simulink model "Model2_V032_R_T4"  (R2023a)
settings: Solver=ode14x  StartTime=0.0  StopTime=Inf  FixedStep=ts  MaxStep=ts  RelTol=1e-5
values from neighbouring files (symbols this model uses):
  ausrollen_a_v = parameters.ausrollen_a_v    [efficiencycalc.m]    (also in parameters_initials.mat = 1)
  bremspunkte = parameters.bremspunkte    [efficiencycalc.m]    (also in parameters_initials.mat = [6100  280  8; 10400  500  3; 14100  550  8; 17729  0  1])
  brennstoffzellen_eta_kennfeld = parameters.brennstoffzellen_eta_kennfeld    [efficiencycalc.m]    (also in parameters_initials.mat = )
  brennstoffzellen_ui_kennfeld = parameters.brennstoffzellen_ui_kennfeld    [efficiencycalc.m]    (also in parameters_initials.mat = )
  coeffs_motor_moment = parameters.coeffs_motor_moment    [efficiencycalc.m]    (also in parameters_initials.mat = [30 30 30 5 7.5 10 0 0 0 6000 6000 6000 ... (30 elements, 3x)
  coeffs_motor_wirkungsgrad = parameters.coeffs_motor_wirkungsgrad    [efficiencycalc.m]    (also in parameters_initials.mat = [30 30 30 5 7.5 10 0 0 0 6000 6000 6000 ... (39 elements, 3x)
  fahrzeug_parameter = parameters.fahrzeug_parameter    [efficiencycalc.m]    (also in parameters_initials.mat = )
  strategie_parameter = parameters.strategie_parameter    [efficiencycalc.m]    (also in parameters_initials.mat = )
  strecke = parameters.strecke    [efficiencycalc.m]    (also in parameters_initials.mat = )
  ts = parameters.ts    [efficiencycalc.m]    (also in parameters_initials.mat = 0.01)
  U_moment = parameters.U_moment    [efficiencycalc.m]    (also in parameters_initials.mat = [30 3])
  U_wirkungsgrad = parameters.U_wirkungsgrad    [efficiencycalc.m]    (also in parameters_initials.mat = [30 3])
  umwelt_parameter = parameters.umwelt_parameter    [efficiencycalc.m]    (also in parameters_initials.mat = )
  zwangsgas = zeros(length(strecke.x),strecke.Rundenzahl)    [Automatisierung_Model_2.m]    (also in efficiencycalc.m; parameters_initials.mat = [0 0 0 0 0 0 0 0 0 0 0 0 ... (2563 elements, 233x11)])
libraries: simulink x1
(part 2 of 3)

== matlab function Model2_V032_R_T4/Energieversorgung/aktueller Ladestatus ==
  data: A_Status input; C_SC input; brennstoffzellen_ui_kennfeld_koeff input; brennstoffzellen_ui_kennfeld_min input; brennstoffzellen_ui_kennfeld_max input; end_charge_Zeitpuffer input; U_SC_initial input; U_SC input; A_Status_neu output; U_SC_min input; t_ges_zul input; Zeit input; ts input; Ladezeit output; v input; x_rest input; ende_bz_an input
function [ A_Status_neu , Ladezeit ]= fcn( A_Status , C_SC, brennstoffzellen_ui_kennfeld_koeff , brennstoffzellen_ui_kennfeld_min , brennstoffzellen_ui_kennfeld_max , end_charge_Zeitpuffer , U_SC_initial , U_SC, U_SC_min, t_ges_zul, Zeit , ts, v, x_rest , ende_bz_an)
%% Aktueller Ladestatus
% Hydro2Motion
% Prototyp: Homer
% Stand: 23.01.2020
% edited: Timo Freilinger

%% Eingang
% A_Status:                                 [-]     alter Status (aus vorherigem Zeitschritt): 0 nicht laden, 1 laden
% C_SC:                                     [F]     Kapazität der SuperCaps
% brennstoffzellen_ui_kennfeld_koeff:       [-]     Koeffizienten des Polynoms, welches Strom aus aktueller Spannung bestimmt
% brennstoffzellen_ui_kennfeld_min:         [V]     untere Spannungsgrenze, ab welcher das Polynom gültig ist
% brennstoffzellen_ui_kennfeld_max:         [V]     obere Spannungsgrenze, bis welcher das Polynom gültig ist
% end_charge_Zeitpuffer:                    [sec]   Zeitpuffer, um am Ende des Rennens früher als nötig begonnen wird, die SC auf Anfangsniveau zu laden (= Zeitunterschied zu Gesamtzeit, die erlaubt ist)
% U_SC_initial:                             [V]     Spannung SC zu Beginn des Rennens (= Spannung, welche am Ende des Rennens wieder vorhanden sein muss)
% U_SC:                                     [V]     aktuelle Spannung SC
% U_SC_min:                                 [V]     in fahrzeug_parameter festgelegte untere Grenze der Spannung SC
% t_ges_zul:                                [sec]   zulässige Gesamtzeit des Rennens
% Zeit:                                     [sec]   aktuelle Simulationszeit
% ts:                                       [sec]   Zeitintervall Berechnung
% v:                                        [m/s]   akt. Geschwindigkeit
% x_rest:                                   [m]     verbleibende Strecke


%% Ausgang
% A_Status_neu:                             [-]     neuer Status (1: Laden, 0: nicht Laden)
% Ladezeit:                                 [sec]   näherungsweise berechnete Zeit, die benötigt wird, um die SC von U_SC (aktuell) auf U_SC_initial zu laden (angenommen, es wird in dieser Zeit nicht zusätzlich Leistung entnommen)

%% Berechnung

%% Initialisierung
A_Status_neu = 0;
Ladezeit = 0;
delta_U = 0;
I_charge = 0;

%% Zeit, die zum Aufladen auf U_SC_initial benötigt werden würde
U_SC_help = U_SC;                                                                                   % U_SC_help: "Hilfsspannung", welche Aufladung symbolisiert
while U_SC_help <= U_SC_initial                                                                     % solange die Spannung kleiner als U_SC_initial ist
    % Berechnung aktueller Ladestrom aus aktueller Spannung (hilf)
    if U_SC_help < brennstoffzellen_ui_kennfeld_min                                            % wenn die aktuelle Spannung (hilf) kleiner als die untere Grenze des Polynoms ist
        I_charge = polyval(brennstoffzellen_ui_kennfeld_koeff,brennstoffzellen_ui_kennfeld_min);     % verwende die untere Grenze des Polynoms als Spannung zur Berechnung des Stroms
    elseif U_SC_help > brennstoffzellen_ui_kennfeld_max                                        % wenn die aktuelle Spannung (hilf) größer als die untere Grenze des Polynoms ist
        I_charge = polyval(brennstoffzellen_ui_kennfeld_koeff,brennstoffzellen_ui_kennfeld_max);     % verwende die obere Grenze des Polynoms als Spannung zur Berechnung des Stroms
    else                                                                                            % ansonsten
        I_charge = polyval(brennstoffzellen_ui_kennfeld_koeff,U_SC_help);                                 % verwende die aktuelle Spannung (hilf) zur Auswertung des Polynoms
    end
    % delta Spannung aus gerade vorliegendem Ladestrom berechnen
    delta_U = I_charge * 10 * ts / C_SC;                                                            % 10, da nur Annäherung! Es wird also angenommen, dass mit dem aktuellen Ladestrom 10*ts geladen wird (Diskretisierung).
    % neue Spannung (hilf) aus alter und delta berechnen
    U_SC_help = U_SC_help + delta_U;
    % Berechnung Ladezeit
    if Zeit ~= 0
        Ladezeit = Ladezeit + 10 * ts;
    end
end

%% Abfrage ob wegen Ende der Strecke nachgeladen wird
% Verbleibende Strecke --> Zeit berechnen mit akt. Geschwindigkeit --> mit
% Ladezeit vergleichen

% v = x / t --> t = x / v
if v > 0
    if x_rest / v - end_charge_Zeitpuffer <= Ladezeit                % Es wird geladen, sobald die restliche Zeit (mit Zeitpuffer) bis ins Ziel kleinergleich der benötigten Ladezeit ist
        A_Status_neu = 1;
    end
end

%% Einschalten BZ
% nach Kriterien:
if A_Status == 0 && U_SC < U_SC_min                              % Unterschreiten der unteren Grenze während Entladung
    A_Status_neu = 1;
elseif U_SC > U_SC_initial                                       % Überschreiten der oberen Grenze
    A_Status_neu = 0;
elseif A_Status == 1 && U_SC > U_SC_min && U_SC < U_SC_initial   % weiter Laden, wenn zwischen Grenzen und geladen wird
    A_Status_neu = 1;
elseif A_Status == 1 && U_SC < U_SC_min                          % falls das unmögliche möglich wird... (so hoher Spannungsabfall, dass kein Berechnungsschritt zwischen oberer und unterer Grenze)
    A_Status_neu = 1;
end

if ende_bz_an == 1
    A_Status_neu = 1;
end
end

== matlab function Model2_V032_R_T4/Energieversorgung/aktueller Ladestrom ==
  data: brennstoffzellen_ui_kennfeld_koeff input; brennstoffzellen_ui_kennfeld_min input; brennstoffzellen_ui_kennfeld_max input; U_SC input; I_charge output; A_Status input
function I_charge = fcn( brennstoffzellen_ui_kennfeld_koeff , brennstoffzellen_ui_kennfeld_min , brennstoffzellen_ui_kennfeld_max , U_SC , A_Status )
%% Aktueller Ladestrom
% Hydro2Motion
% Prototyp: Homer
% Stand: 23.01.2020
% edited: Timo Freilinger

%% Eingang
% brennstoffzellen_ui_kennfeld_koeff:       [-]     Koeffizienten des Polynoms, welches Strom aus aktueller Spannung bestimmt
% brennstoffzellen_ui_kennfeld_min:         [V]     untere Spannungsgrenze, ab welcher das Polynom gültig ist
% brennstoffzellen_ui_kennfeld_max:         [V]     obere Spannungsgrenze, bis welcher das Polynom gültig ist
% U_SC:                                     [V]     aktuelle Spannung SC
% A_Status:                                 [-]     aktueller Ladestatus (1: Laden, 0: nicht Laden)

%% Ausgang
% I_charge:                                 [A]     aktueller Ladestrom

%% Berechnung

% Initialisierung, bzw. Ladestrom, wenn nicht geladen wird
I_charge = 0;
% wenn geladen wird
if A_Status == 1
    % prüfen, ob aktuelle Spannung außerhalb der für das Polynom verwendeten Grezen liegt
    if U_SC > brennstoffzellen_ui_kennfeld_max                 % wenn die aktuelle Spannung größer als die obere Grenze des Polynoms ist
        U_SC = brennstoffzellen_ui_kennfeld_max;               % verwende die obere Grenze des Polynoms als Spannung zur Berechnung des Stroms
    elseif U_SC < brennstoffzellen_ui_kennfeld_min             % wenn die aktuelle Spannung kleiner als die untere Grenze des Polynoms ist
        U_SC = brennstoffzellen_ui_kennfeld_min;               % verwende die untere Grenze des Polynoms als Spannung zur Berechnung des Stroms
    end
    % berechne aktuellen Ladestrom, abhängig von der aktuellen Spannung
    I_charge = polyval(brennstoffzellen_ui_kennfeld_koeff, U_SC);
end

end

== matlab function Model2_V032_R_T4/Energieversorgung/Berechnung delta Spannung Aufladung ==
  data: I_charge input; ts input; C_SC input; delta_U_SC_charge output; t input
function delta_U_SC_charge = fcn( I_charge , ts , C_SC , t )
%% Berechnung delta Spannung Aufladung
% Hydro2Motion
% Prototyp: Homer
% Stand: 23.01.2020
% edited: Timo Freilinger

%% Eingang
% I_charge:             [A]     aktueller Ladestrom
% ts:                   [sec]   Zeitintervall Berechnung
% C_SC:                 [F]     Kapazität der Kondensatoren
% t:                    [sec]   aktuelle Simulationszeit

%% Ausgang
% delta_U_SC_charge:    [V]     aktuelle Spannungsdifferenz, mit der SC aufgeladen werden

%% Berechnung

if t == 0                                        % Initialisierung zu Beginn der Simulation
    delta_U_SC_charge = 0;
elseif I_charge == 0                             % wenn kein Ladestrom vorhanden
    delta_U_SC_charge = 0;                       % wird nicht geladen
else                                             % wenn Ladestrom vorhanden
    delta_U_SC_charge = I_charge * ts / C_SC;    % Spannungsdifferenz berechnen
end

end

== matlab function Model2_V032_R_T4/Fahr-Dynamik/Widerstände über Kennzahlen/Berechnung Luftwiderstand ==
  data: rho_0 input; F_L output; v input; cw_A input
function F_L = fcn(rho_0,v,cw_A)
%% Besrechnung Luftwiderstand
% Hydro2Motion
% Prototyp: Homer
% Stand: 04.01.2018
% edited: Robin Nedella, Timo Freilinger

%% Eingang
% rho_0:    [kg/m^3]    Luftdichte
% v:        [m/s]       aktuelle Geschwindigkeit
% cw_A:     [m^2]       Strömungswiderstandsfläche

%% Ausgabe
% F_L:      [N]         Luftwiderstandskraft

%% Berechnung
F_L = rho_0 / 2 * v^2 * cw_A;   % [N]

end

== matlab function Model2_V032_R_T4/Fahr-Dynamik/Widerstände über Kennzahlen/Berechnung Rollwiderstand ==
  data: f_roll input; F_R output; m_ges input; g input; steigung input; v input; hoehenradius input
function F_R = fcn(f_roll,m_ges,g,steigung,v,hoehenradius)
%% Berechnung Rollwiderstand
% Hydro2Motion
% Prototyp: Homer
% Stand: 06.01.2019
% edited: Robin Nedella, Timo Freilinger

%% Eingang
% f_roll: Rollwiderstandsbeiwert
% m_ges: gesamte Masse
% g: Erdbeschleunigung
% steigung: aktuelle Steigung [rad]
% v: aktuelle Geschwindigkeit

%% Ausgabe
% F_R: Rollwiderstandskraft

%% Berechnung
% Rollwiderstands_Gain, um bei Null Geschwindigkeit keine Kraft entgegen Fahrrichtung zu haben
v_umsch = 0.05;              % Umschaltgeschwindigkeit in m/s, ab der auf "realen" Rollwiderstand geschalten wird
if abs(v) < v_umsch
    Rollwiderstands_Gain = v / v_umsch;
else
    Rollwiderstands_Gain = 1;
end
Rollwiderstands_Gain = Rollwiderstands_Gain * sign ( v );           % Sicherheit vor Rückwärtsrollen (Rollwiderstand wechselt Richtung)

F_R = f_roll * m_ges * (g * cos(steigung) + v^2/hoehenradius) * Rollwiderstands_Gain;   % [N]

end

== matlab function Model2_V032_R_T4/Energieversorgung/Berechnung aktueller Wirkungsgrad Brennstoffzelle ==
  data: I_charge input; U_SC input; brennstoffzellen_eta_kennfeld_koeff input; eta_bz_aktuell output; brennstoffzellen_eta_kennfeld_min input; brennstoffzellen_eta_kennfeld_max input
function eta_bz_aktuell = fcn( I_charge , U_SC , brennstoffzellen_eta_kennfeld_koeff , brennstoffzellen_eta_kennfeld_min , brennstoffzellen_eta_kennfeld_max )
%% Aktueller Wirkungsgrad Brennstoffzelle
% Hydro2Motion
% Prototyp: Homer
% Stand: 23.01.2020
% edited: Timo Freilinger

%% Eingang
% I_charge:                          [A]     aktueller Ladestrom 
% U_SC:                              [V]     aktuelle SC-Spannung
% brennstoffzellen_eta_kennfeld:     [-]     Koeffizienten des Polynoms BZ-Wirkungsgrad
% brennstoffzellen_eta_kennfeld_min: [V]     untere Grenze der Spannung, bei welcher das Polynom korrekt berechnet wird
% brennstoffzellen_eta_kennfeld_max: [V]     obere Grenze der Spannung, bei welcher das Polynom korrekt berechnet wird

%% Ausgang
% eta_bz_aktuell:                    [-]     aktueller Wirkungsgrad Brennstoffzelle

%% Berechnung

U_SC_eta = U_SC;                                 % "Initialisierung"

if U_SC < brennstoffzellen_eta_kennfeld_min         % wenn die aktuelle Spannung kleiner als die untere Grenze des Polynoms ist
    U_SC_eta = brennstoffzellen_eta_kennfeld_min;   % verwende die untere Grenze des Polynoms als Spannung zur Berechnung des Wirkungsgrades
elseif U_SC > brennstoffzellen_eta_kennfeld_max     % wenn die aktuelle Spannung größer als die obere Grenze des Polynoms ist
    U_SC_eta = brennstoffzellen_eta_kennfeld_max;   % verwende die obere Grenze des Polynoms als Spannung zur Berechnung des Wirkungsgrades
end

% Wirkungsgrad anhand aktueller Spannung und Polynom berechnen
eta_bz_aktuell = polyval(brennstoffzellen_eta_kennfeld_koeff, U_SC_eta);

% wenn aktuell nicht geladen wird
if I_charge == 0
    eta_bz_aktuell = 1;     % Wirkungsgrad auf "1" gesetzt, damit später nicht durch Null dividiert wird
end

end

== matlab function Model2_V032_R_T4/Fahr-Dynamik/MATLAB Function ==
  data: J_standard input; J_ges output; J_antrieb input; fps input
function J_ges = fcn(J_standard,J_antrieb,fps)
%% Berechnung Gesamtträgheitsmoment
% Hydro2Motion
% Prototyp: Homer
% Stand: 23.01.2020
% edited: Robin Nedella

%% Eingang
% J_standard: Standard-Trägheit, welche immer vorhanden ist
% J_antrieb: Antrieb-Trägheit, welche nur bei aktivem Motor vorhanden ist
% fps: Fahrpedalstellung

%% Ausgang
% J_ges: gesamte Trägheit aller im aktuellen Zustand rotierenden Teile

%% Berechnung
if fps == 0                             % falls kein Gas gegeben wird
    J_ges = J_standard;                     % ist die gesamte Trägheit gleich der Standard-Trägheit
else                                    % falls Gas gegeben wird
    J_ges = J_standard + J_antrieb;         % wird zur Standard-Trägheit die Antriebs-Trägheit addiert
end

end

== matlab function Model2_V032_R_T4/Energieversorgung/neue Spannung SC berechnen ==
  data: U_SC_initial input; U_SC input; delta_U_SC_discharge input; U_SC_neu output; delta_U_SC_charge input; t input
function U_SC_neu = fcn( U_SC_initial , U_SC , delta_U_SC_discharge , delta_U_SC_charge , t )
%% neue SC-Spannung berechnen
% Hydro2Motion
% Prototyp: Homer
% Stand: 23.01.2020
% edited: Timo Freilinger

%% Eingang
% U_SC:                     [V]     aktuelle SC Spannung
% delta_U_SC_discharge:     [V]     delta Entladung
% delta_U_SC_charge:        [V]     delta Beladung
% t:                        [sec]   aktuelle Simulationszeit

%% Ausgang
% U_SC_neu:              neue SC Spannung

%% Berechnung

if t == 0                                                           % zu Beginn der Simulation 
    U_SC_neu = U_SC_initial;                                        % ist Spannung SC initial
else                                                                % während der Simulation
    U_SC_neu = U_SC + delta_U_SC_charge + delta_U_SC_discharge;     % neue Spannung = alte + Beladung - Entladung (trotzdem "+", da Vorzeichen zuvor richtig berechnet)
end

end

== matlab function Model2_V032_R_T4/Energieversorgung/Initialisierung SuperCaps Spannung ==
  data: clock input; U_SC1 output; U_SC input; U_SC_initial input
function U_SC1 = fcn(clock,U_SC,U_SC_initial)
%% Initialisierung SuperCaps Spannung
% Hydro2Motion
% Prototyp: Homer
% Stand: 23.01.2020
% edited: Timo Freilinger

%% Eingang
% clock         [sec]   aktuelle Simulationszeit
% U_SC          [V]     aktuelle Spannung der SuperCaps
% U_SC_initial  [V]     Spannung der SuperCaps zu Beginn der Simulation

%% Ausgang
% U_SC1         [V]     aktuelle Spannung der SuperCaps

%% Berechnung
% da Simulink intern zu Beginn der Simulation noch unbekannte Variablen auf Null setzt:

U_SC1 = U_SC;
% Damit keine "Warnung", dass durch Null geteilt (bei t=0)
if clock == 0
    U_SC1 = U_SC_initial;
end

end

== matlab function Model2_V032_R_T4/Energieversorgung/Berechnung delta Spannung Entladung sekundär ==
  data: U_SC input; P_sekundaer input; delta_U_SC_discharge_sekundaer output; C_SC input; ts input; t input; P_Luefter input; A_Status input
function delta_U_SC_discharge_sekundaer = fcn( U_SC , P_sekundaer , C_SC , ts , t, P_Luefter, A_Status )
%% Berechnung Entladung durch Sekundärverbräuche
% Hydro2Motion
% Prototyp: Homer
% Stand: 23.01.2020
% edited: Timo Freilinger

%% Eingang
% U_SC:                             [V]     aktuelle Spannung SuperCaps
% P_sekundaer:                      [W]     Sekundärverbräuche
% C_SC:                             [F]     Kapazität der SuperCaps
% ts:                               [sec]   Zeitschritt der Berechnung
% t:                                [sec]   Berechnungszeit der Simulation
% P_Luefter:                        [W]     Leistung des BZ Lüfters inkl.
% Ventile 
% A_Status:                         [-]     Status der BZ

%% Ausgang
% delta_U_SC_discharge_sekundaer:  Betrag der Spannung, um welchen die SC aktuell entladen werden

%% Berechnung
% Berechnung Entladestrom durch Sekundärverbräuche
if A_Status == 0
    % BZ aus
    I = P_sekundaer / U_SC;
else
    % BZ an
    I = (P_sekundaer + P_Luefter) / U_SC;
end

if t == 0                                    % initial zu Beginn der Simulation
    delta_U_SC_discharge_sekundaer = 0;                % werden die SC nicht entladen
else                                         % ansonsten werden die SC entladen
    delta_U_SC_discharge_sekundaer = - I * ts / C_SC;  % Spannungsabfall der SC im Simulationsschritt ts
end

end

== matlab function Model2_V032_R_T4/Fahr-Dynamik/Berechnung Kurvenwiderstand ==
  data: F_K output; m_ges input; v input; radius input; c_alpha input
function F_K = fcn(m_ges,v,radius,c_alpha)
%% Berechnung Kurvenwiderstand
% Hydro2Motion
% Prototyp: Homer
% Stand: 23.01.2020
% edited: Robin Nedella

%% Eingang
% m_ges:        gesamte Masse
% v:            aktuelle Geschwindigkeit
% radius:       aktueller Kurvenradius
% c_alpha:      Schraeglaufsteifgkeiten der Raeder (aus H2M Handbuch)

%% Ausgabe
% F_K: Kurvenwiderstandskraft

%% Berechnung Kurvenwiderstandskraft

F_K = (0.5 * m_ges^2 * v^4) / (c_alpha *  radius^2);   % [N]

end

== matlab function Model2_V032_R_T4/Fahr-Dynamik/Berechnung Steigungswiderstand ==
  data: F_S output; m_ges input; g input; steigung input
function F_S = fcn(m_ges,g,steigung)
%% Berechnung Steigungswiderstand
% Hydro2Motion
% Prototyp: Homer
% Stand: 23.01.2020
% edited: Robin Nedella

%% Eingang
% m_ges: gesamte Masse
% g: Erdbeschleunigung
% steigung: aktuelle Steigung [rad]

%% Ausgabe
% F_S: Steigungswiderstandskraft

%% Berechnung
F_S = m_ges * g * sin(steigung);   % [N]

end

== matlab function Model2_V032_R_T4/Fahrer // Strategie/MATLAB Function ==
  data: v input; v_alt input; v_durch input; bremskraft output; position_runde input; bremspunkte input; distanz_3d input; bremskraft_max input; wegpunkt input; delta_s output; ignore_bremse_alt input; ignore_bremse output
function [bremskraft, delta_s, ignore_bremse]= fcn(v, v_alt,  v_durch, position_runde, bremspunkte, distanz_3d, bremskraft_max, wegpunkt, ignore_bremse_alt )
%% Bremsfunktion
% Hydro2Motion
% Prototyp: Homer
% Stand: 23.01.2020
% edited: Timo Freilinger

bremskraft = 0;
delta_s = 0;
ignore_bremse = 0;

i = 1;

%% Nächsten Bremspunkt aus Strecke ermitteln
while (position_runde >= bremspunkte(i))
    i = i + 1;
    if i >= length(bremspunkte)
        % erster Punkt der Nächsten Runde
        i = 1;
        break;
    end
end

next_bremspunkt = bremspunkte(i,1);
abstand_bremsbeginn = bremspunkte(i,2);  % xxx m vor der Stillhaltestelle Bremsen beginnen
brems_gain = bremspunkte(i,3);

if (next_bremspunkt >= position_runde) 
    % Nächster Bremspunkt in aktueller Runde
    delta_s = next_bremspunkt - position_runde ;
else
    % Nächster Bremspunkt in nächster Runde
    delta_s = distanz_3d(end) - position_runde + bremspunkte(1,1);
end

% wenn v +-20m null wird, kann wieder normal Gas gegeben werden.
if delta_s < abstand_bremsbeginn
    bremskraft =  brems_gain * delta_s * bremskraft_max / abstand_bremsbeginn + 0.1;
end

if delta_s < 20 && v <= 0
    bremskraft = 0;
end

if v_alt > 0 && v <= 0
    ignore_bremse = 1;
end

if ignore_bremse_alt == 1
    if v >= v_durch
        ignore_bremse = 0;
    else
        bremskraft = 0;
        ignore_bremse = 1;
    end
end

end

== matlab function Model2_V032_R_T4/Fahrer // Strategie/Entscheidung ueber Simulationsende ==
  data: fertige_runden input; ende output; runde_sim input; v_gain output; fps_gain output; U_SC input; U_SC_initial input; v input; bz_status output
function [ ende , v_gain , fps_gain , bz_status]= fcn( fertige_runden , runde_sim , U_SC , U_SC_initial , v)
%% Simulationsende
% Hydro2Motion
% Prototyp: Homer
% Stand: 23.01.2020
% edited: Robin Nedella

%% Eingang
% fertige_runden:    Anzahl der bereits absolvierten Runden
% runde_sim:         Zahl der zu simulierenden Runden
% U_SC:              aktuelle Spannung der SuperCaps
% U_SC_initial:      zu Beginn des Rennens vorliegende Spannung in den SC --> Muss am Ende des Rennens wieder auf diesem Niveau liegen!

%% Ausgang
% ende:              0: weiter simulieren, 1: Stop der Simulation
% v_gain:            1: Auto noch nicht im Ziel, keine Beeinflussung, 0: Auto im Ziel --> keine Geschwindigkeit
% fps_gain:          1: Auto noch nicht im Ziel, keine Beeinflussung, 0: Auto im Ziel --> kein Gas mehr

%% Berechnung
% Initialisierung
ende = 0;
v_gain = 1;
fps_gain = 1;
bz_status = 0;

% Ende Simulation, wenn Gesamtstrecke erreicht UND SC auf Anfangsspannung
if fertige_runden >= runde_sim      % dann ist Ziel erreicht
    v_gain = 0;                         % keine Geschwindigkeit mehr
    fps_gain = 0;                       % nicht mehr Gas geben
    bz_status = 1;
    if U_SC >= U_SC_initial             % wenn zudem aktuelle SC-Spannung auf Anfangsniveau liegt
        ende = 1;                           % Ende der Simulation
    end
end

% Abbruch, wenn Auto stehen bleibt
if v < 0
    ende = 1;
end

end

== matlab function Model2_V032_R_T4/Fahrer // Strategie/SuperCaps-Spannung berücksichtigen ==
  data: fps_neu input; fps output; k_n input; U_SC input; MC_max_voltage_gain input; n_motor input; n_motor_max output; ignore_rollen input; Spannungslimit_alt input; Spannungslimit output; U_Motor output; F_brems input
function [fps , n_motor_max, Spannungslimit, U_Motor]= fcn( fps_neu , k_n , U_SC ,  MC_max_voltage_gain,  n_motor, ignore_rollen, Spannungslimit_alt, F_brems)
%% SuperCaps-Spannung berücksichtigen
% Hydro2Motion
% Prototyp: Homer
% Stand: 23.01.2020
% edited: Robin Nedella

%% Eingang
% fps_neu:                  [-]         durch Strategie und Zwangsgas vorgegebene fps (0: kein Gas, 1: Gas)
% k_n:                      [rps/V]     Drehzahlkonstante Motor
% U_SC:                     [V]         aktuelle Spannung in den SuperCaps
% MC_max_voltage_gain:      [-]         Quotient aus Aus- und Eingangsspannung Motorcontroller, was maximal möglich ist
% n_motor:                  [rps]       aktuelle Motordrehzahl, wenn im aktuellen Berechnungsschritt Gas gegeben werden würde

%% Ausgang
% fps:                      [-]         kommandierte Fahrpedalstellung
% n_motor_max               [rps]       maximal mögliche Motordrehzahl unter Berücksichtigung der SC-Spannung

%% Berechnung
% Beachtung der SuperCaps-Spannung
% DAS HAT OBERSTEN VORRANG !!

    % Initialisierung
Spannungslimit = Spannungslimit_alt;    % Spanungslimit aus vorherigem Zeitschritt
fps            = fps_neu;               % durch Strategie und Zwangsgas vorgegebene fps (0: kein Gas, 1: Gas)

    % Berechnung der maximal möglichen Motordrehzahl bei aktueller SC-Spannung
n_motor_max = k_n * U_SC * MC_max_voltage_gain;

    % vom Motor benötigte Spannung
U_Motor = n_motor / k_n;

    % [V] oberer Mindestabstand zur oberen Grenze der max. möglichen Drehzahl
delta_U1 = 0.1;
    % [V] unterer Mindestabstand zur oberen Grenze der max. möglichen Drehzahl, bis wieder Gas gegeben wird
delta_U2 = 6;

    % wenn oberer Mindestabstand unterschritten
if (U_SC * MC_max_voltage_gain - delta_U1) <=  U_Motor 
        fps = 0;
        Spannungslimit = 1;
end
 
    % wenn oberer Mindestabstand im vorangegangenen Zeitschritt unterschritten
if Spannungslimit_alt == 1
        % wenn unterer Mindestabstand unterschritten
    if (U_SC * MC_max_voltage_gain - U_Motor) > delta_U2
            % Unterdrückung Gas geben aufgehoben
        Spannungslimit = 0;
        
        % wenn unterer Mindestabstand noch nicht unterschritten
    else
            % weiterhin Unterdrückung Gas geben
        Spannungslimit = 1;
    end
end


% Kein Gas, wenn Motordrehzahl zu nah an der maximal möglichen liegt
if Spannungslimit == 1
    fps = 0;
end

%% für Bremsen zusätzlich nötig:
if ignore_rollen == 1
    fps = 1;
elseif n_motor > n_motor_max
    fps = 0;
end

if F_brems > 0
    fps = 0;
end

end

== matlab function Model2_V032_R_T4/Fahrer // Strategie/Kurvenüberwachung ==
  data: fps_last input; Strecke_Radius input; v input; wegpunkt input; distanz_3d input; Gas_Kurve output; min_gas_zeit input; crit_radius_gas input; min_Radius input
function Gas_Kurve = fcn( fps_last , Strecke_Radius, v , wegpunkt , distanz_3d , min_gas_zeit , crit_radius_gas , min_Radius )
%% Kurvenüberwachung
% Hydro2Motion
% Prototyp: Homer
% Stand: 23.01.2020
% edited: Robin Nedella

%% Eingänge
% fps_last:        FPS des vorherigen Zeitschritts
% Strecke_Radius:  Vektor mit Strecken Radius Daten
% v:               aktuelle Geschwindigkeit
% wegpunkt:        aktueller Wegpunkt
% distanz_3d:      Distanz 3D
% min_gas_zeit:    Zeit, die mindestens am Stück vor der Kurve (oder auf der Geraden) Gas gegeben werden können muss
% crit_radius_gas: Radius, unter dem kein Gas mehr gegeben werden darf

%% Ausgänge
% Gas_kurve: 1, wenn Gas ok, 0, wenn zu nah an nächster Kurve

%% Berechnung
% Initialisierung
Gas_Kurve = 1;

%% Weg zur nächsten Kurve bestimmen
% nächster Radius
r_next = Strecke_Radius(wegpunkt);
% aktueller Wegpunkt
next_curve = wegpunkt;
% geht die Streckenmatrix nach vorne durch, bis die nächste enge Kurve gefunden wird
if min_Radius < crit_radius_gas % zur Überprüfung, um zu verhindern, dass es keinen Kurvenradius gibt, der kleiner als der kritische ist (sonst: Endlos-Schleife in der Berechnung)
    if crit_radius_gas ~= 0
        while r_next > crit_radius_gas                   % solange Radius größer als minimaler, bis zu welchem Gas gegeben werden darf (crit_radius_gas)
            if next_curve < length(Strecke_Radius)    % wenn erfüllt, dann liegt aktuell betrachteter Wegpunkt nicht am Ende der Streckenmatrix
                % Nächster Wegpunkt
                next_curve = next_curve + 1;
            else                                         % wenn Ende der Runde erreicht, zähle am Anfang der Strecke weiter
                % Strecke beginnt wieder von vorne
                next_curve = next_curve + 1 - length(Strecke_Radius);
            end
            % nimmt den Radius einen Wegpunkt weiter
            r_next = Strecke_Radius(next_curve);
        end
        %% Überschlagsmäßige Berechnung der Zeit für diesen Weg (ohne Fahrwiderstände)
        delta_weg = 0;                                                                     % Initialisierung
        if next_curve >= wegpunkt                                                          % Abfrage, ob nächste Kurve noch in aktueller Runde
            % nächste Kurve liegt vor dem Ende der aktuellen Runde
            delta_weg = distanz_3d(next_curve) - distanz_3d(wegpunkt);                     % Weg zwischen aktuellem Wegpunkt und der nächsten Kurve
        else
            % beginnt die Strecke wieder von Vorne
            delta_weg = distanz_3d(end) - distanz_3d(wegpunkt) + distanz_3d(next_curve);   % Weg zwischen aktuellem Wegpunkt und der nächsten Kurve
        end
        % Zeit bis zur nächsten Kurve mit aktueller Geschwindigkeit überschlagen (Annahme: aktuelle Geschwindigkeit wird bis zur nächsten Kurve gehalten)
        delta_zeit = delta_weg / v;                                                        % näherungsweise Konstante Geschwindigkeit bis zur nächsten Kurve

        % Entscheiden, ob die Zeit lange genug ist, um noch Gas zu geben
        if delta_zeit <= min_gas_zeit
            % Wenn zu nah an Kurve --> kein Gas
            Gas_Kurve = 0;
        end
        % wenn davor Gas gegeben wird, weiterhin Gas geben
        if fps_last == 1 && Gas_Kurve == 0 && Strecke_Radius(wegpunkt) > crit_radius_gas
            Gas_Kurve = 1;
        end
    end
end

end

== matlab function Model2_V032_R_T4/Motorsteuerung/Bestimmung des tatsächlichen Stroms ==
  data: I output; I_max input; fps input; time input
function I = fcn( I_max , fps , time)
%% Bestimmung des tatsächlichen Stroms
% Hydro2Motion
% Prototyp: Homer
% Stand: 23.01.2020
% edited: Robin Nedella

%% Eingang
% I_max:         [A]     durch Strategie-Parameter maximal möglicher Strom
% fps:           [-]     Fahrpedalstellung
% time:          [s]     Simulationszeit

%% Ausgang
% I:             [A]     tatsächlicher Strom

%% Berechnung

if fps == 0   % wenn kein Gas gegeben wird
    I = 0;      % wird kein Strom benötigt
else          % wenn Gas gegeben wird
    % Wenn allgemein mit sehr geringem vorgegebenem Strom gefahren wird,
    % dann kann hier für bestimmte Zeit am Anfang mehr Strom gegeben
    % werden, um den Anfahrvorgang besser zu bestreiten.
    if time < 50  % für eine bestimmte Zeit am Anfang des Rennens
        I = 10;       % wird mehr Strom gegeben
    else % wenn die Anfanhrzeit vorüber ist und Gas gegeben wird
        I = I_max;  % Strom auf den durch Strategie erlaubten begrenzt
    end
    I = I_max;  % dann ist der gefahrene Strom gleich dem in den Strategie_Parametern hinterlegte
end

end

== matlab function Model2_V032_R_T4/Motorsteuerung/Bestimmung_Moment_aus_Polynomen ==
  data: M_U_up output; I input; M_motor output; U_SC input; n_motor input; M_U_down output; U_moment input; coeffs_motor_moment input; M_U_down_I_down output; M_U_down_I_up output; M_U_up_I_down output; M_U_up_I_up output; k_M input
function [ M_U_up , M_motor , M_U_down , M_U_down_I_down , M_U_down_I_up , M_U_up_I_down , M_U_up_I_up ] = fcn( I , U_SC , n_motor , U_moment , coeffs_motor_moment , k_M )
%% Bestimmung Moment aus Polynomen
% Hydro2Motion
% Prototyp: Homer
% Stand: 23.01.2020
% edited: Robin Nedella

%% Eingang
% I:                        [A]     aktuell gefahrener Strom
% U_SC:                     [V]     aktuelle Spannung in den SuperCaps, also aktuelle Spannung am Motorcontroller
% n_motor:                  [rps]   aktuelle Motordrehzahl
% coeffs_motor_moment:      []      Matrix, in welcher die Koeffizienten der Polynome hinterlegt sind (Spalte 1: Strom, 2: Spanung, ab 3: Koeffizienten)
% U_moment:                 [V]     Vektor, in welchem die Spannungen stehen, welche in coeffs hinterlegt

%% Ausgang
% M_motor:                [-]     aktueller Moment Motor bei aktuellem Strom und aktueller Spannung
% M_U_down:               [-]     aktueller Moment Motor bei nächst kleinerem Strom und aktueller Spannung
% M_U_up:                 [-]     aktueller Moment Motor bei nächst größerem Strom und aktueller Spannung

%%
n_motor = n_motor * 60; % Polynome basieren auf RPM, nicht RPS

%% Initialisierung
U_down = 0; % nächst kleinere Spannung, für welche Polynome hinterlegt
U_up = 0;   % nächst größere Spannung, für welche Polynome hinterlegt

U_down_I_down = 0; % nächst kleinerer Strom für untere Spannung, für welchen Polynom hinterlegt
U_up_I_down = 0;   % nächst kleinerer Strom für obere Spannung, für welchen Polynom hinterlegt
U_down_I_up = 0;   % nächst größerer Strom für untere Spannung, für welchen Polynom hinterlegt
U_up_I_up = 0;     % nächst größerer Strom für obere Spannung, für welchen Polynom hinterlegt

I_U_down = zeros(1,2);
I_U_up = zeros(1,2);

row_U_down_I_down = 0;  % Zeile, in welcher Koeffizienten für nächst kleineren Strom und nächst kleineren Spannung steht
row_U_down_I_up = 0;    % Zeile, in welcher Koeffizienten für nächst kleineren Strom und nächst größeren Spannung steht
row_U_up_I_down = 0;    % Zeile, in welcher Koeffizienten für nächst größeren Strom und nächst kleineren Spannung steht
row_U_up_I_up = 0;      % Zeile, in welcher Koeffizienten für nächst größeren Strom und nächst größerer Spannung steht

n_motor_U_down_I_down = 0;  % Motordrehzahl, mit welcher das Polynom ausgewertet wird (Gültigkeitsbereich Polynom beachtet) nächst kleinere Spannung und nächst kleinerer Strom
n_motor_U_down_I_up = 0;    % Motordrehzahl, mit welcher das Polynom ausgewertet wird (Gültigkeitsbereich Polynom beachtet) nächst kleinere Spannung und nächst größerer Strom
n_motor_U_up_I_down = 0;    % Motordrehzahl, mit welcher das Polynom ausgewertet wird (Gültigkeitsbereich Polynom beachtet) nächst größere Spannung und nächst kleinerer Strom
n_motor_U_up_I_up = 0;      % Motordrehzahl, mit welcher das Polynom ausgewertet wird (Gültigkeitsbereich Polynom beachtet) nächst größere Spannung und nächst größerer Strom

M_U_down_I_down = 0;  % aktuelles Motormoment bei nächst kleinerer Spannung und nächst kleinerem Strom
M_U_down_I_up = 0;    % aktuelles Motormoment bei nächst kleinerer Spannung und nächst größerem Strom
M_U_up_I_down = 0;    % aktuelles Motormoment bei nächst größerer Spannung und nächst kleinerem Strom
M_U_up_I_up = 0;      % aktuelles Motormoment bei nächst größerer Spannung und nächst größerem Strom

M_U_down = 0;         % aktuelles Motormoment bei nächst kleinerer Spannung und aktuellem Strom
M_U_up = 0;           % aktuelles Motormoment bei nächst größerer Spannung und aktuellem Strom

M_motor = 0;          % aktuelles Motormoment bei aktuellem Strom und aktueller Spannung (hier: Initialisierung)
%%
if I ~= 0   % wenn gleich null, dann M_motor = 0 (es muss nichts berechnet werden)
    
    %% suche 2 nächsten Spannungen
        % wenn unter kleinster: nimm kleinste Spannung
    if U_SC < U_moment(1,1)       % wenn aktuelle Spannung kleiner als kleinste im KF hinterlegte
        U_down = U_moment(1,1);       % nächst kleinere Spannung ist kleinste hinterlegte Spannung
        U_up = U_moment(1,1);         % nächst größere Spannung ist kleinste hinterlegte Spannung
        I_U_down = zeros(U_moment(1,2),2);       % Initialisierung des Vektors, wo Ströme, welche bei nächst kleinerer Spannung im Kennfeld hinterlegt sind, gespeichert werden
        I_U_up = zeros(U_moment(1,2),2);         % Initialisierung des Vektors, wo Ströme, welche bei nächst größerer Spannung im Kennfeld hinterlegt sind, gespeichert werden

    elseif U_SC > U_moment(end,1) % wenn aktuelle Spannung größer als größte im KF hinterlegte
        U_down = U_moment(end,1);     % nächst kleinere Spannung ist größte hinterlegte Spannung
        U_up = U_moment(end,1);       % nächst größere Spannung ist größte hinterlegte Spannung
        I_U_down = zeros(U_moment(end,2),2);       % Initialisierung des Vektors, wo Ströme, welche bei nächst kleinerer Spannung im Kennfeld hinterlegt sind, gespeichert werden
        I_U_up = zeros(U_moment(end,2),2);         % Initialisierung des Vektors, wo Ströme, welche bei nächst größerer Spannung im Kennfeld hinterlegt sind, gespeichert werden
    else                                % dann liegt aktuelle Spannung an den Grenzen der m KF hinterlegten Spannungen oder dazwischen
        j = 2;                        % Initialisierung, sonst error
        for j = 1:1:length(U_moment)  % prüfe, ob die gefahrene Spannung direkt im KF hinterlegt ist
           if U_SC == U_moment(j)         % wenn die gefahrene Spannung direkt im KF hinterlegt ist
               U_down = U_SC;                       % dann muss nicht interpoliert werden
               U_up = U_SC;
               I_U_down = zeros(U_moment(j,2),2);       % Initialisierung des Vektors, wo Ströme, welche bei nächst kleinerer Spannung im Kennfeld hinterlegt sind, gespeichert werden
               I_U_up = zeros(U_moment(j,2),2);         % Initialisierung des Vektors, wo Ströme, welche bei nächst größerer Spannung im Kennfeld hinterlegt sind, gespeichert werden
               break;
           elseif U_SC < U_moment(j)      % ansonsten: finde die beiden im Kennfeld hinterlegten Spannungen, zwischen welchen die gefahrene Spannung liegt
               U_down = U_moment(j-1);        % Spannung im Kennfeld, welche am nächsten auf kleineren Seite an die gefahrene Spannung kommt
               U_up = U_moment(j);            % Spannung im Kennfeld, welche am nächsten auf größerer Seite an die gefahrene Spannung kommt
               I_U_down = zeros(U_moment(j-1,2),2);       % Initialisierung des Vektors, wo Ströme, welche bei nächst kleinerer Spannung im Kennfeld hinterlegt sind, gespeichert werden
               I_U_up = zeros(U_moment(j,2),2);         % Initialisierung des Vektors, wo Ströme, welche bei nächst größerer Spannung im Kennfeld hinterlegt sind, gespeichert werden
               break;
           end
        end
    end
    
    %% speichere jeweils die hinterlegten Ströme; 1. Spalte: in welcher Zeile von coeffs_motor_moment steht der Strom; 2. Spalte: Strom
         % für untere Spannung (I_U_down)
    j = 2;                        % Initialisierung, sonst error
    for j = 1:1:length(coeffs_motor_moment(:,1))
        if coeffs_motor_moment(j,1) == U_down
            k = j;
            m = 1;
            while coeffs_motor_moment(k,1) == U_down
                I_U_down(m,2) = coeffs_motor_moment(k,2);
                I_U_down(m,1) = k;
                m = m + 1;
                k = k + 1;
                if k > length(coeffs_motor_moment(:,1))    % dann steht in der nächsten Zeile nicht mehr U_down
                    break;
                end
            end
            break;
        end        
    end
        % für obere Spannung (I_U_up)
    j = 2;                        % Initialisierung, sonst error
    for j = 1:1:length(coeffs_motor_moment(:,1))
        if coeffs_motor_moment(j,1) == U_up
            k = j;
            m = 1;
            while coeffs_motor_moment(k,1) == U_up
                I_U_up(m,2) = coeffs_motor_moment(k,2);   % 2. Spalte: Strom
                I_U_up(m,1) = k;                                % 1. Spalte: Zeile aus coeffs_motor_Moment, in welcher der Strom steht
                m = m + 1;
                k = k + 1;
                if k > length(coeffs_motor_moment(:,1))    % dann steht in der nächsten Zeile nicht mehr U_up
                    break;
                end
            end
            break;
        end        
    end
    
    %% suche für untere und obere Spannung jeweils die 2 nächsten Ströme und speichere die Zeile, wo sie in coeffs_motor_Moment zu finden sind
        %% untere Spannung
    if I < I_U_down(1,2) || I > I_U_down(end,2)
       M_U_down = I * k_M;          % keine Vermessung hinterlegt --> Berechnung aus Drehmomentenkonstante
    else                            % KF hinterlegt bzw Interpolation möglich
        j = 2;                        % Initialisierung, sonst error
        for j = 1:1:length(I_U_down)
          if I == I_U_down(j,2)                 % wenn gefahrene Strom dirket im Kennfeld hinterlegt ist
              row_U_down_I_down = I_U_down(j,1);
              row_U_down_I_up = I_U_down(j,1);
              U_down_I_down = I_U_down(j,2);
              U_down_I_up = I_U_down(j,2);
              break;
          elseif I < I_U_down(j,2)
              row_U_down_I_down = I_U_down(j-1,1);
              row_U_down_I_up = I_U_down(j,1);
              U_down_I_down = I_U_down(j-1,2);
              U_down_I_up = I_U_down(j,2);
              break;
          end
        end
        % Gültigkeitsbereich beachten
            % Motordrehzahl, mit welcher Polynom für nächst kleinere Spannung und nächst kleinerem Strom ausgewertet wird
        if n_motor < coeffs_motor_moment(row_U_down_I_down,3)
            n_motor_U_down_I_down = coeffs_motor_moment(row_U_down_I_down,3);
        elseif n_motor > coeffs_motor_moment(row_U_down_I_down,4)
            n_motor_U_down_I_down = coeffs_motor_moment(row_U_down_I_down,4);
        else
            n_motor_U_down_I_down = n_motor;
        end
            % Motordrehzahl, mit welcher Polynom für nächst kleinere Spannung und nächst größerem Strom ausgewertet wird
        if n_motor < coeffs_motor_moment(row_U_down_I_up,3)
            n_motor_U_down_I_up = coeffs_motor_moment(row_U_down_I_up,3);
        elseif n_motor > coeffs_motor_moment(row_U_down_I_up,4)
            n_motor_U_down_I_up = coeffs_motor_moment(row_U_down_I_up,4);
        else
            n_motor_U_down_I_up = n_motor;
        end
        % Berechnung: Auswertung des Polynoms
            % aktueller Moment für nächst kleineren Strom bei nächst kleinerer Spannung
        M_U_down_I_down = polyval( fliplr( coeffs_motor_moment( row_U_down_I_down , 5:end )) , n_motor_U_down_I_down);
            % aktueller Moment für nächst größeren Strom bei nächst kleinerer Spannung
        M_U_down_I_up   = polyval( fliplr( coeffs_motor_moment( row_U_down_I_up   , 5:end )) , n_motor_U_down_I_up);
        % Interpolation zwischen Strömen
            % interpolierter Moment des aktuellen Stroms bei nächst kleinerer Spannung
        if U_down_I_down == U_down_I_up         % dann muss nicht interpoliert werden
            M_U_down = M_U_down_I_down;         % nimm eta_U_down_I_down oder eta_U_down_I_up
        else                                    % dann muss interpoliert werden
            M_U_down = (I - U_down_I_down) * (M_U_down_I_up - M_U_down_I_down) / (U_down_I_up - U_down_I_down) + M_U_down_I_down;
        end
    end
        %% obere Spannung
    if I < I_U_up(1,2) || I > I_U_up(end,2)
       M_U_up = I * k_M;
    else
        j = 2;                        % Initialisierung, sonst error
        for j = 1:1:length(I_U_up)
          if I == I_U_up(j,2)                 % wenn gefahrene Strom dirket im Kennfeld hinterlegt ist
              row_U_up_I_down = I_U_up(j,1);
              row_U_up_I_up = I_U_up(j,1);
              U_up_I_down = I_U_up(j,2);
              U_up_I_up = I_U_up(j,2);
              break;
          elseif I < I_U_up(j,2)
              row_U_up_I_down = I_U_up(j-1,1);
              row_U_up_I_up = I_U_up(j,1);
              U_up_I_down = I_U_up(j-1,2);
              U_up_I_up = I_U_up(j,2);
              break;
          end
        end
        % Gültigkeitsbereich beachten
            % Motordrehzahl, mit welcher Polynom für nächst größere Spannung und nächst kleinerem Strom ausgewertet wird
        if n_motor < coeffs_motor_moment(row_U_up_I_down,3)
            n_motor_U_up_I_down = coeffs_motor_moment(row_U_up_I_down,3);
        elseif n_motor > coeffs_motor_moment(row_U_up_I_down,4)
            n_motor_U_up_I_down = coeffs_motor_moment(row_U_up_I_down,4);
        else
            n_motor_U_up_I_down = n_motor;
        end
                % Motordrehzahl, mit welcher Polynom für nächst größere Spannung und nächst größerem Strom ausgewertet wird
        if n_motor < coeffs_motor_moment(row_U_up_I_up,3)
            n_motor_U_up_I_up = coeffs_motor_moment(row_U_up_I_up,3);
        elseif n_motor > coeffs_motor_moment(row_U_up_I_up,4)
            n_motor_U_up_I_up = coeffs_motor_moment(row_U_up_I_up,4);
        else
            n_motor_U_up_I_up = n_motor;
        end
        % Berechnung
            % aktueller Moment für nächst kleineren Strom bei nächst größerer Spannung
        M_U_up_I_down   = polyval( fliplr( coeffs_motor_moment( row_U_up_I_down   , 5:end )) , n_motor_U_up_I_down);
            % aktueller Moment für nächst kleineren Strom bei nächst kleinerer Spannung
        M_U_up_I_up     = polyval( fliplr( coeffs_motor_moment( row_U_up_I_up     , 5:end )) , n_motor_U_up_I_up);
        % Interpolation zwischen Strömen
            % interpoliere Moment des aktuellen Stroms bei nächst größerer Spannung
        if U_up_I_down == U_up_I_up             % dann muss nicht interpoliert werden
            M_U_up = M_U_up_I_down;             % nimm eta_U_up_I_down oder eta_U_up_I_up
        else                                    % dann muss interpoliert werden
            M_U_up   = (I - U_up_I_down)   * (M_U_up_I_up   - M_U_up_I_down)   / (U_up_I_up   - U_up_I_down)   + M_U_up_I_down;
        end
    end
    
    %% Interpoliere zwischen den Spannungen dann linear
        % wenn udown = uup dann keine interpolation nötig
    if U_down == U_up                       % dann muss nicht interpoliert werden
        M_motor = M_U_down;                 % nimm eta_U_down oder eta_U_up
    else
        M_motor = (U_SC - U_down) * (M_U_up - M_U_down) / (U_up - U_down) + M_U_down;
    end
    
    %% Umrechnung auf [Nm]
    M_motor = M_motor / 1000;
end

end

== matlab function Model2_V032_R_T4/Motorsteuerung/Kennfeld MC und Motor separat/MATLAB Function ==
  data: P_Motor_out input; P_Motor_in output; n_motor input; coeff_motor_wirkungsgrad input; eta_Motor output
function [P_Motor_in , eta_Motor]= fcn(P_Motor_out , n_motor , coeff_motor_wirkungsgrad)
% Hydro2Motion
% Prototyp: Homer
% Stand: 23.01.2020
% edited: Robin Nedella

%% Bestimmung aktueller Motorwirkungsgrad
% Code um aus Koeffizienten der Wirkungsgradkurve und der Drehzahl den eta_Motor zu berechnen
eta_Motor = 1;

%% Bestimmung benötigte Leistung
% Berechnung Leistung, die vom MC an Motor abgegeben werden muss
P_Motor_in = P_Motor_out / eta_Motor;   % Berechnung Leistung, welche in Motor geht

end

== matlab function Model2_V032_R_T4/Motorsteuerung/Kennfeld MC und Motor separat/MATLAB Function2 ==
  data: P_Motor_in input; P_MC_in output; U_SC input; coeff_MC_wirkungsgrad input
function P_MC_in = fcn(P_Motor_in , U_SC , coeff_MC_wirkungsgrad)
% Hydro2Motion
% Prototyp: Homer
% Stand: 23.01.2020
% edited: Robin Nedella

%% Bestimmung aktueller Motorwirkungsgrad
% Code um aus Koeffizienten der Wirkungsgradkurve und der Drehzahl den eta_Motor zu berechnen
eta_MC = 1;

%% Bestimmung benötigte Leistung
% Berechnung Leistung, die vom MC an Motor abgegeben werden muss
P_MC_out = P_Motor_in;            % vom MC abgegebene Leistung entspricht der in den Motor gehenden Leistung
P_MC_in = P_MC_out / eta_MC;   % Berechnung Leistung, welche in Motor geht


end
